simulink model "Aufgabe5"  (R2015b)
settings: Solver=VariableStepAuto  StartTime=0.0  StopTime=10.0  RelTol=1e-3
values from neighbouring files (symbols this model uses):
  A = A_tablle(i)    [Aufgabe5_script.m]
  B = B_tablle(i)    [Aufgabe5_script.m]
  C = C_tablle(i)    [Aufgabe5_script.m]
settings Model: Creator=lukaskiechle  LastModifiedBy=lukaskiechle

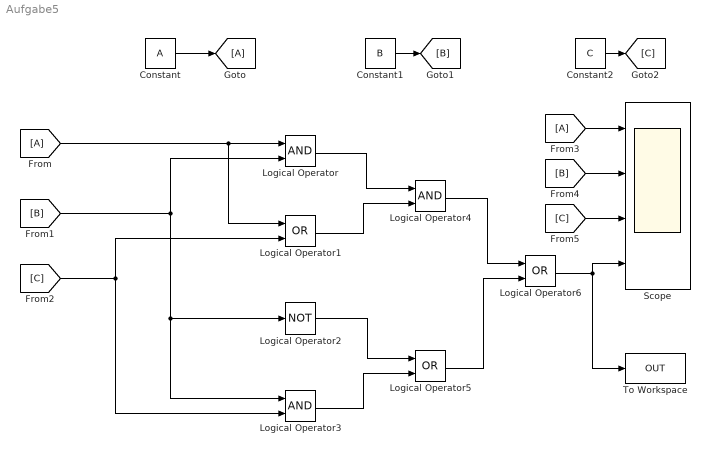
== system Aufgabe5 ==
  Constant : Constant  Value=A
  Constant1 : Constant  Value=B
  Constant2 : Constant  Value=C
  Logical Operator : Logic  AllPortsSameDT=off  OutDataTypeStr=boolean
  Logical Operator1 : Logic  Operator=OR  AllPortsSameDT=off  OutDataTypeStr=boolean
  Logical Operator2 : Logic  Operator=NOT  Inputs=1  AllPortsSameDT=off  OutDataTypeStr=boolean
  Logical Operator3 : Logic  AllPortsSameDT=off  OutDataTypeStr=boolean
  Logical Operator4 : Logic  AllPortsSameDT=off  OutDataTypeStr=boolean
  Logical Operator5 : Logic  Operator=OR  AllPortsSameDT=off  OutDataTypeStr=boolean
  Logical Operator6 : Logic  Operator=OR  AllPortsSameDT=off  OutDataTypeStr=boolean
  Scope : Scope  NumInputPorts=4
  To Workspace : ToWorkspace  VariableName=OUT  SampleTime=-1
  wires:
  Logical Operator/1 -> Logical Operator4/1
  Logical Operator1/1 -> Logical Operator4/2
  Logical Operator2/1 -> Logical Operator5/1
  Logical Operator3/1 -> Logical Operator5/2
  Logical Operator4/1 -> Logical Operator6/1
  Logical Operator5/1 -> Logical Operator6/2
  Logical Operator6/1 -> To Workspace/1, Scope/4
  Constant1/1 -> [B]
  Constant2/1 -> [C]
  Constant/1 -> [A]
  [A] -> Logical Operator1/1, Logical Operator/1
  [B] -> Logical Operator/2, Logical Operator2/1, Logical Operator3/1
  [C] -> Logical Operator1/2, Logical Operator3/2
  [A] -> Scope/1
  [B] -> Scope/2
  [C] -> Scope/3
